simulink model "Demo_MPC"  (R2020a)
settings: Solver=VariableStepAuto  StartTime=0.0  StopTime=10.0  RelTol=1e-3
settings Model: Creator=86150  LastModifiedBy=86150

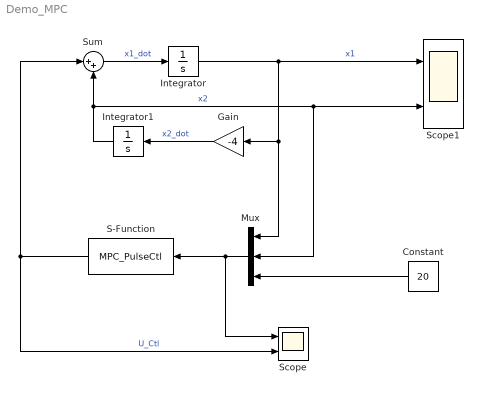
== system Demo_MPC ==
  Constant : Constant  Value=20
  Gain : Gain  Gain=-4
  Integrator : Integrator
  Integrator1 : Integrator
  Mux : Mux  Inputs=3
  S-Function : S-Function  FunctionName=MPC_PulseCtl  SFunctionDeploymentMode=off  EnableBusSupport=off
  Scope : Scope  NumInputPorts=2
  Scope1 : Scope  NumInputPorts=2
  Sum : Sum  Inputs=|++
  wires:
  Mux/1 -> Scope/1, S-Function/1
  Constant/1 -> Mux/3
  S-Function/1 -> Scope/2, Sum/1  "U_Ctl"
  Sum/1 -> Integrator/1  "x1_dot"
  Integrator/1 -> Mux/1, Gain/1, Scope1/1  "x1"
  Gain/1 -> Integrator1/1  "x2_dot"
  Integrator1/1 -> Mux/2, Scope1/2, Sum/2  "x2"
